simulink model "Final_EWASP_VC"  (R2022a)
settings: Solver=ode1  StartTime=0.0  StopTime=24*3600  FixedStep=10  RelTol=1e-3
values from neighbouring files (symbols this model uses):
  Aux_Threshold = 52    [Setup_Code_EWASP_VC.m]
  buildingAge = 2005    [Setup_Code_EWASP_VC.m]
  ceilingHeight = 2.4    [Setup_Code_EWASP_VC.m]
  conductiveHconnectMatrix = [ ... (first row only)    [Setup_Code_EWASP_VC.m]
  cRoofGreen = 100000    [Setup_Code_EWASP_VC.m]
  Defrost_After_Time = 30    [Setup_Code_EWASP_VC.m]
  DHWDemandProfile = occFreegainHotwaterElecTestPassiveOcc3(:,3)    [Setup_Code_EWASP_VC.m]
  Elec_Max = Elec_Max*(30/24.2)    [Setup_Code_EWASP_VC.m]
  Elec_Mid = Elec_Mid*(30/24.2)    [Setup_Code_EWASP_VC.m]
  Elec_Min = Elec_Min*(30/24.2)    [Setup_Code_EWASP_VC.m]
  ElecDemandProfile = occFreegainHotwaterElecTestPassiveOcc3(:,4)    [Setup_Code_EWASP_VC.m]
  ElecFixed = [Elec_Max(6,2) Elec_Max(6,4) Elec_Max(6,6) Elec_Max(6,7) ... (first row only)    [Setup_Code_EWASP_VC.m]
  floorOrCeilingArea = floorOrCeilingArea*1.15    [Setup_Code_EWASP_VC.m]
  forceCold = 0    [Setup_Code_EWASP_VC.m]
  freegain = occFreegainHotwaterElecTestPassiveOcc3(:,2)-max(occupancy)*25    [Setup_Code_EWASP_VC.m]
  furnitureModelOn = 1    [Setup_Code_EWASP_VC.m]
  Heat_Max = Heat_Max*(30/24.2)    [Setup_Code_EWASP_VC.m]
  Heat_Mid = Heat_Mid*(30/24.2)    [Setup_Code_EWASP_VC.m]
  Heat_Min = Heat_Min*(30/24.2)    [Setup_Code_EWASP_VC.m]
  HeatFixed = [Heat_Max(6,2) Heat_Max(6,4) Heat_Max(6,6) Heat_Max(6,7) ... (first row only)    [Setup_Code_EWASP_VC.m]
  HeatingOnProfile = repmat(HeatingOnProfile,365,1)    [Setup_Code_EWASP_VC.m]
  HEX_ReturnLowerLimit = 52.5    [Setup_Code_EWASP_VC.m]
  HEX_ReturnUpperLimit = 55    [Setup_Code_EWASP_VC.m]
  LeakMultiplier = 1+(2*(rand()-0.5)/10)    [Setup_Code_EWASP_VC.m]
  loopCap = 15    [Setup_Code_EWASP_VC.m]
  maxOcc = max(occupancyProfile)    [Setup_Code_EWASP_VC.m]
  NESW_wallArea = max(NESW_Lengths*ceilingHeight-NESW_Windows,0)    [Setup_Code_EWASP_VC.m]
  NESW_Windows = [ ... (first row only)    [Setup_Code_EWASP_VC.m]
  numRooms = roomCount    [Setup_Code_EWASP_VC.m]
  offsetDays = 0    [Setup_Code_EWASP_VC.m]
  pumpChoice = pumpChoices(MinIndex,1)    [Setup_Code_EWASP_VC.m]
  pumpRamp = 180    [Setup_Code_EWASP_VC.m]
  ReturnLowerLimit = 37.5    [Setup_Code_EWASP_VC.m]
  ReturnUpperLimit = 40    [Setup_Code_EWASP_VC.m]
  RoofIrradiance = Flat_NS_EW_RoofIrradiance(:,1)    [Setup_Code_EWASP_VC.m]
  roofStartTemp = ones(11,1)*20    [Setup_Code_EWASP_VC.m]
  rooftype = 0    [Setup_Code_EWASP_VC.m]
  RoomDataMatrix = [zeros(1,12);ones(1,12)*wallDensity;zeros(1,12);ones(1,12)*wallU;ones(1,12)*windowU;ones(1,12)*floorU;ones(1,12)*ceilingU;zeros(1,12);windowArea, 0;floorOrCeilingArea;zeros(1,12);floorOrCeilingArea*ceilingHeight]    [Setup_Code_EWASP_VC.m]
  roomVol = roomVol*1.15    [Setup_Code_EWASP_VC.m]
  slabStartTemp = (GroundTempTimeSeries(offsetDays*1440+1,1)+thermostatSetting)/2    [Setup_Code_EWASP_VC.m]
  SlackRequest = zeros(1440,1)    [Setup_Code_EWASP_VC.m]
  SolarThermalExists = 0    [Setup_Code_EWASP_VC.m]
  SourceFixed = HeatFixed-ElecFixed    [Setup_Code_EWASP_VC.m]
  StateSeries = StateSeriesGenerator(22,7,1)    [Setup_Code_EWASP_VC.m]
  Tank_Lower_Temp = 49.5    [Setup_Code_EWASP_VC.m]
  Tank_Upper_Temp = 52    [Setup_Code_EWASP_VC.m]
  Tank_Volume_m3 = 0.15    [Setup_Code_EWASP_VC.m]
  TankHeatHour = randi([1 5])-1    [Setup_Code_EWASP_VC.m]
  thermostatSetting = 20.0    (= 20)    [Setup_Code_EWASP_VC.m]
  upDown = [0;0;0;0;1;1;1;1;1;1;1]    [Setup_Code_EWASP_VC.m]
  variableASHP = 1    [Setup_Code_EWASP_VC.m]
  wallStartTempExt = thermostatSetting*(0.266+0.00215*outdoorStartTemp+0.018*wallU+0.00113*outdoorStartTemp*wallU+0.0068*wallU^2)    [Setup_Code_EWASP_VC.m]
undefined symbols (not defined in the file or in its folder): a, ceilingU, condUDMatrix, convUDMatrix, deltaPEXPANDED_E, deltaPEXPANDED_E2, deltaPEXPANDED_N, deltaPEXPANDED_N2, deltaPEXPANDED_S, deltaPEXPANDED_S2, deltaPEXPANDED_W, deltaPEXPANDED_W2, DesiredDHWTemp, DesiredFlowTempVsInOutDeltaTemp, DiffuseHorizontal, DiscIntNeverNeededParam, DNI, dwnAndConcrete, DWORK_A_HX, DWORK_CHK_FLU, DWORK_CP_NODE, DWORK_DH, DWORK_FLUID, DWORK_HCON, DWORK_LOSS, DWORK_MDOTDOWN, DWORK_MDOTIN, DWORK_MDOTUP, DWORK_MIX, DWORK_PRESS, DWORK_QDOTIN, DWORK_RHO_NODE, DWORK_TIN, DWORK_TS_OLD, DWORK_V_NODE, GroundTempTimeSeries, HCM, HCM2, HCM_closed, HCM_closed2, intermediateU, IsTop, massFlowMatrix, neighbourMatrix, numericalRoomUse, RadiatorMatrix, room2roomflowmatrix_E, room2roomflowmatrix_E2, room2roomflowmatrix_N, room2roomflowmatrix_N2, room2roomflowmatrix_S, room2roomflowmatrix_S2, room2roomflowmatrix_W, room2roomflowmatrix_W2, StateAirInEXPANDED_E, StateAirInEXPANDED_E2, StateAirInEXPANDED_N, StateAirInEXPANDED_N2, StateAirInEXPANDED_S, StateAirInEXPANDED_S2 ... (+23)
libraries: simulink x6, dspsigops x4, dspmtrx3 x4, carnot x3, spsEdgeDetectorLib x2, dspstat3 x2, powerlib_meascontrol x1, simulink_extras x1
(part 2 of 27)

== system Final_EWASP_VC/GSHP_Subsystem ==
  note: Monitors for debugging
  Constant3 : Constant  Value=3600
  DHW for GSHP case : Subsystem
  Delay6 : Delay  DelayLength=5  InitialCondition=0
  Discrete-Time Integrator1 : DiscreteIntegrator  ExternalReset=falling  SampleTime=-1  LimitOutput=on  UpperSaturationLimit=1  LowerSaturationLimit=0  ICPrevOutput=DiscIntNeverNeededParam  ICPrevScaledInput=DiscIntNeverNeededParam
  Divide1 : Product  Inputs=*/
  Divide2 : Product  Inputs=*/
  Integrator14 : Integrator
  IsInf : RelationalOperator  Operator=isNaN  OutDataTypeStr=boolean  RndMeth=Simplest  InputSameDT=off
  Massflow when system is on12 : Constant  Value=3400/3600
  Plus : Sum
  Product : Product
  Product1 : Product
  Product3 : Product  Inputs=*/
  Scope21 : Scope
  Subsystem3 : Subsystem
      mask Display:
      | port_label('input', 1, 'T_Out')
      | port_label('input', 2, 'MixedTemp')
      | port_label('input', 3, 'MassFlowTotal')
      | port_label('input', 4, 'GCS')
      | port_label('input', 5, 'PowerFraction')
      | port_label('input', 6, 'DHW_on')
      | port_label('input', 7, 'ToGroundTot')
      | 
      | port_label('output', 1, 'Hysteresis')
      | port_label('output', 2, 'd_signal')
      | port_label('output', 3, 'THB_to_Pre')
      | 
      | port_label('output', 4, 'HeatToSpace')
      | port_label('output', 5, 'ElectrifiedHeatToSpace')
      | port_label('output', 6, 'ToGround')
      | port_label('output', 7, 'TotMdot')
      | 
      | disp('SH_GSHP')
  Sum : Sum  Inputs=|++
  Sum7 : Sum  Inputs=|++
  Switch2 : Switch  Criteria=u2 > Threshold  Threshold=0.5  SaturateOnIntegerOverflow=off  InputSameDT=off
  T_mains : Constant  Value=12
  Time in seconds for Heat pump to reach full stady state output1 : Constant  Value=180
  Water Demand Time Series (Minute)1 : Constant  Value=DHWDemandProfile
  tank_sensor_temp : Scope
  tag scope: AuxHeatToWater=global, DHW_on=global, ElectrifiedHeatToSpaceG=global, ElectrifiedHeatToWater=global, HeatToSpace=global, HeatToWater=global, THB_In_Pre=global, ToGround2=global, ToGround=global, ToGroundTot=global, TotMdot2=global, TotMdot=global, d_signal=global, d_signal_DHW=global, hysteresis=global, pump_power_Fraction=global
  wires:
  Product3/1 -> Switch2/3, IsInf/1
  Water Demand Time Series (Minute)1/1 -> DHW for GSHP case/5(In5)
  Subsystem3/4(Out4) -> [HeatToSpace]
  Integrator14/1 -> Scope21/1
  Divide2/1 -> Discrete-Time Integrator1/1
  DHW for GSHP case/1(Out1) -> tank_sensor_temp/1
  [d_signal] -> Plus/1
  DHW for GSHP case/2(Out2) -> [DHW_on]
  [MassFlowTotal] -> Subsystem3/3(In3)
  [DHW_on] -> Subsystem3/6(In6)
  [T_Out] -> Subsystem3/1(In1)
  DHW for GSHP case/7(Out7) -> [AuxHeatToWater]
  Discrete-Time Integrator1/1 -> Delay6/1
  [ToGround] -> Switch2/1, Product/1
  DHW for GSHP case/6(Out6) -> [HeatToWater]
  Subsystem3/3(Out3) -> [THB_In_Pre]
  [MixedTemp] -> Subsystem3/2(In2)
  Subsystem3/1(Out1) -> [hysteresis]
  [FromGround] -> DHW for GSHP case/1(In1)
  Plus/1 -> Divide2/1, Discrete-Time Integrator1/2
  Time in seconds for Heat pump to reach full stady state output1/1 -> Divide2/2
  [ToGround2] -> Product1/1
  [HeatToSpace] -> Divide1/1
  DHW for GSHP case/3(Out3) -> [ToGround2]
  [d_signal_DHW] -> Plus/2
  DHW for GSHP case/5(Out5) -> [ElectrifiedHeatToWater]
  Delay6/1 -> [pump_power_Fraction]
  Divide1/1 -> Integrator14/1
  [TotMdot] -> Product/2, Sum/1
  Product/1 -> Sum7/1
  DHW for GSHP case/4(Out4) -> [TotMdot2]
  Constant3/1 -> Divide1/2
  Subsystem3/7(Out7) -> [TotMdot]
  Massflow when system is on12/1 -> DHW for GSHP case/6(In6)
  DHW for GSHP case/8(Out8) -> [d_signal_DHW]
  [pump_power_Fraction] -> Subsystem3/5(In5)
  Subsystem3/6(Out6) -> [ToGround]
  Subsystem3/5(Out5) -> [ElectrifiedHeatToSpaceG]
  [ToGroundTot] -> Subsystem3/7(In7)
  Subsystem3/2(Out2) -> [d_signal]
  [Global_Control_Signal] -> Subsystem3/4(In4)
  [TotMdot2] -> Product1/2, Sum/2
  Sum/1 -> Product3/2
  [T_Out] -> DHW for GSHP case/3(In3)
  Product1/1 -> Sum7/2
  Sum7/1 -> Product3/1
  T_mains/1 -> DHW for GSHP case/4(In4)
  IsInf/1 -> Switch2/2
  Switch2/1 -> [ToGroundTot]
  [T_1] -> DHW for GSHP case/2(In2)
  Subsystem3/8(Out8) -> [FromGround]

== system Final_EWASP_VC/Offset Independent time series element selector ==
  In1 : Inport
  Clock1 : Clock
  Direct Lookup Table (n-D)1 : LookupNDDirect  NumberOfTableDimensions=1  TableIsInput=on
  Divide1 : Product  Inputs=*/
  Floor : Rounding
  Saturation2 : Saturate  UpperLimit=inf  LowerLimit=0
  Scope23 : Scope
  Sum : Sum  Inputs=|++
  on? (I/O)1 : Constant  Value=0  OutDataTypeStr=double
  on? (I/O)3 : Constant  Value=60  OutDataTypeStr=double
  Out1 : Outport  VectorParamsAs1DForOutWhenUnconnected=off
  wires:
  Saturation2/1 -> Scope23/1, Direct Lookup Table (n-D)1/1
  on? (I/O)3/1 -> Divide1/2
  Divide1/1 -> Floor/1
  Floor/1 -> Saturation2/1
  Clock1/1 -> Sum/1
  Direct Lookup Table (n-D)1/1 -> Out1/1
  In1/1 -> Direct Lookup Table (n-D)1/2
  on? (I/O)1/1 -> Sum/2
  Sum/1 -> Divide1/1

== system Final_EWASP_VC/Offset Independent time series element selector1 ==
  In1 : Inport
  Clock1 : Clock
  Direct Lookup Table (n-D)1 : LookupNDDirect  NumberOfTableDimensions=1  TableIsInput=on
  Divide1 : Product  Inputs=*/
  Floor : Rounding
  Saturation2 : Saturate  UpperLimit=inf  LowerLimit=0
  Scope23 : Scope
  Sum : Sum  Inputs=|++
  on? (I/O)2 : Constant  Value=offsetDays*3600*24  OutDataTypeStr=double
  on? (I/O)3 : Constant  Value=60  OutDataTypeStr=double
  Out1 : Outport  VectorParamsAs1DForOutWhenUnconnected=off
  wires:
  Saturation2/1 -> Scope23/1, Direct Lookup Table (n-D)1/1
  on? (I/O)3/1 -> Divide1/2
  Divide1/1 -> Floor/1
  Floor/1 -> Saturation2/1
  Clock1/1 -> Sum/1
  Direct Lookup Table (n-D)1/1 -> Out1/1
  In1/1 -> Direct Lookup Table (n-D)1/2
  Sum/1 -> Divide1/1
  on? (I/O)2/1 -> Sum/2

== system Final_EWASP_VC/Offset Independent time series element selector2 ==
  In1 : Inport
  Clock1 : Clock
  Direct Lookup Table (n-D)1 : LookupNDDirect  NumberOfTableDimensions=1  TableIsInput=on
  Divide1 : Product  Inputs=*/
  Floor : Rounding
  Saturation2 : Saturate  UpperLimit=inf  LowerLimit=0
  Scope23 : Scope
  Sum : Sum  Inputs=|++
  on? (I/O)1 : Constant  Value=0  OutDataTypeStr=double
  on? (I/O)3 : Constant  Value=60  OutDataTypeStr=double
  Out1 : Outport  VectorParamsAs1DForOutWhenUnconnected=off
  wires:
  Saturation2/1 -> Scope23/1, Direct Lookup Table (n-D)1/1
  on? (I/O)3/1 -> Divide1/2
  Divide1/1 -> Floor/1
  Floor/1 -> Saturation2/1
  Clock1/1 -> Sum/1
  Direct Lookup Table (n-D)1/1 -> Out1/1
  In1/1 -> Direct Lookup Table (n-D)1/2
  on? (I/O)1/1 -> Sum/2
  Sum/1 -> Divide1/1

== system Final_EWASP_VC/Radiator w//Thermostatic Control ==
  In1 : Inport
  In2 : Inport  Port=2
  In3 : Inport  Port=3
  1/(m*cp) : Gain  Gain=1/(Water_Volume*4180)  SaturateOnIntegerOverflow=on  OutDataTypeStr=Inherit: Same as input  ParamDataTypeStr=Inherit: Same as input
  Abs : Abs
  Add : Sum  Inputs=+-
  Constant : Constant  Value=4181
  Constant1 : Constant  Value=TRV_Therm_Setpoint
  Constant2 : Constant  Value=0.5
  Discrete-Time Integrator : DiscreteIntegrator  SampleTime=-1  ICPrevOutput=DiscIntNeverNeededParam  ICPrevScaledInput=DiscIntNeverNeededParam
  Divide : Product  Inputs=*/
  Divide1 : Product  Inputs=**
  Math Function : Math  Operator=pow  SignedPower=on
  Product : Product  Inputs=3  InputSameDT=on  SaturateOnIntegerOverflow=on  OutDataTypeStr=Inherit: Same as first input
  Product1 : Product  InputSameDT=on  SaturateOnIntegerOverflow=on  OutDataTypeStr=Inherit: Same as first input
  Product2 : Product
  Qdot2room1 : Scope
  Saturation : Saturate  UpperLimit=1  LowerLimit=0
  Scope : Scope
  Sign : Signum
  Sum : Sum  Inputs=-+  InputSameDT=on  SaturateOnIntegerOverflow=on  OutDataTypeStr=Inherit: Same as first input
  Sum1 : Sum  Inputs=-+  InputSameDT=on  SaturateOnIntegerOverflow=on  OutDataTypeStr=Inherit: Same as first input
  Sum2 : Sum
  Sum3 : Sum  Inputs=-+  InputSameDT=on  SaturateOnIntegerOverflow=on  OutDataTypeStr=Inherit: Same as first input
  Transfer Fcn (with initial states) : simulink_extras/Additional Linear/Transfer Fcn (with initial states)  Commented=on  N=[1]  D="[1  0]"  X0=20
  const : Constant  Value=1.3
  const1 : Constant  Value=Power_Nominal
  dTnom : Constant  Value=DeltaT_Nominal
  Out1 : Outport  VectorParamsAs1DForOutWhenUnconnected=off
  Out2 : Outport  Port=2  VectorParamsAs1DForOutWhenUnconnected=off
  Out3 : Outport  Port=3  VectorParamsAs1DForOutWhenUnconnected=off
  wires:
  Sum/1 -> Product/1
  Sum1/1 -> 1/(m*cp)/1
  Constant/1 -> Product/3
  Sum3/1 -> Sign/1, Divide/1
  const/1 -> Math Function/2
  Sign/1 -> Product1/2
  Product1/1 -> Out1/1, Sum1/1
  dTnom/1 -> Divide/2
  Abs/1 -> Math Function/1
  Product/1 -> Sum1/2
  In2/1 -> Sum/2
  const1/1 -> Divide1/2
  Divide1/1 -> Product1/1
  1/(m*cp)/1 -> Discrete-Time Integrator/1
  Math Function/1 -> Divide1/1
  Discrete-Time Integrator/1 -> Sum3/2, Sum/1, Scope/1, Out2/1
  Divide/1 -> Abs/1
  In1/1 -> Add/2, Sum3/1
  Product2/1 -> Product/2, Out3/1
  In3/1 -> Product2/1
  Constant1/1 -> Add/1
  Add/1 -> Sum2/1
  Constant2/1 -> Sum2/2
  Sum2/1 -> Saturation/1
  Saturation/1 -> Qdot2room1/1, Product2/2

== system Final_EWASP_VC/Select Correct Element from Array1 ==
  In1 : Inport
  Constant : Constant  Value=60
  Digital Clock : DigitalClock  SampleTime=10
  Direct Lookup Table (n-D) : LookupNDDirect  NumberOfTableDimensions=1  TableIsInput=on
  Divide : Product  Inputs=*/
  Floor : Rounding
  Saturation : Saturate  UpperLimit=inf  LowerLimit=0
  Out1 : Outport  VectorParamsAs1DForOutWhenUnconnected=off
  wires:
  Divide/1 -> Floor/1
  Saturation/1 -> Direct Lookup Table (n-D)/1
  Constant/1 -> Divide/2
  Floor/1 -> Saturation/1
  In1/1 -> Direct Lookup Table (n-D)/2
  Digital Clock/1 -> Divide/1
  Direct Lookup Table (n-D)/1 -> Out1/1

== system Final_EWASP_VC/Select Correct Element from Array2 ==
  In1 : Inport
  Constant : Constant  Value=60
  Digital Clock : DigitalClock  SampleTime=10
  Direct Lookup Table (n-D) : LookupNDDirect  NumberOfTableDimensions=1  TableIsInput=on
  Divide : Product  Inputs=*/
  Floor : Rounding
  Saturation : Saturate  UpperLimit=1439  LowerLimit=0
  Out1 : Outport  VectorParamsAs1DForOutWhenUnconnected=off
  wires:
  Divide/1 -> Floor/1
  Saturation/1 -> Direct Lookup Table (n-D)/1
  Constant/1 -> Divide/2
  Floor/1 -> Saturation/1
  In1/1 -> Direct Lookup Table (n-D)/2
  Digital Clock/1 -> Divide/1
  Direct Lookup Table (n-D)/1 -> Out1/1

== system Final_EWASP_VC/Select correct element from array, considering offset ==
  In1 : Inport
  Clock1 : Clock
  Direct Lookup Table (n-D)1 : LookupNDDirect  NumberOfTableDimensions=1  TableIsInput=on
  Divide1 : Product  Inputs=*/
  Floor : Rounding
  Saturation2 : Saturate  UpperLimit=inf  LowerLimit=0
  Scope23 : Scope
  Sum : Sum  Inputs=|++
  on? (I/O)1 : Constant  Value=offsetDays*3600*24  OutDataTypeStr=double
  on? (I/O)3 : Constant  Value=60  OutDataTypeStr=double
  Out1 : Outport  VectorParamsAs1DForOutWhenUnconnected=off
  wires:
  Saturation2/1 -> Scope23/1, Direct Lookup Table (n-D)1/1
  on? (I/O)3/1 -> Divide1/2
  Divide1/1 -> Floor/1
  Floor/1 -> Saturation2/1
  Clock1/1 -> Sum/1
  Direct Lookup Table (n-D)1/1 -> Out1/1
  In1/1 -> Direct Lookup Table (n-D)1/2
  on? (I/O)1/1 -> Sum/2
  Sum/1 -> Divide1/1

== system Final_EWASP_VC/Select correct element from array, considering offset1 ==
  In1 : Inport
  Clock1 : Clock
  Direct Lookup Table (n-D)1 : LookupNDDirect  NumberOfTableDimensions=1  TableIsInput=on
  Divide1 : Product  Inputs=*/
  Floor : Rounding
  Saturation2 : Saturate  UpperLimit=inf  LowerLimit=0
  Scope23 : Scope
  Sum : Sum  Inputs=|++
  on? (I/O)1 : Constant  Value=offsetDays*3600*24  OutDataTypeStr=double
  on? (I/O)3 : Constant  Value=60  OutDataTypeStr=double
  Out1 : Outport  VectorParamsAs1DForOutWhenUnconnected=off
  wires:
  Saturation2/1 -> Scope23/1, Direct Lookup Table (n-D)1/1
  on? (I/O)3/1 -> Divide1/2
  Divide1/1 -> Floor/1
  Floor/1 -> Saturation2/1
  Clock1/1 -> Sum/1
  Direct Lookup Table (n-D)1/1 -> Out1/1
  In1/1 -> Direct Lookup Table (n-D)1/2
  on? (I/O)1/1 -> Sum/2
  Sum/1 -> Divide1/1

== system Final_EWASP_VC/Select correct element from array, considering offset2 ==
  In1 : Inport
  Clock1 : Clock
  Direct Lookup Table (n-D)1 : LookupNDDirect  NumberOfTableDimensions=1  TableIsInput=on
  Divide1 : Product  Inputs=*/
  Floor : Rounding
  Saturation2 : Saturate  UpperLimit=inf  LowerLimit=0
  Scope23 : Scope
  Sum : Sum  Inputs=|++
  on? (I/O)1 : Constant  Value=offsetDays*3600*24  OutDataTypeStr=double
  on? (I/O)3 : Constant  Value=60  OutDataTypeStr=double
  Out1 : Outport  VectorParamsAs1DForOutWhenUnconnected=off
  wires:
  Saturation2/1 -> Scope23/1, Direct Lookup Table (n-D)1/1
  on? (I/O)3/1 -> Divide1/2
  Divide1/1 -> Floor/1
  Floor/1 -> Saturation2/1
  Clock1/1 -> Sum/1
  Direct Lookup Table (n-D)1/1 -> Out1/1
  In1/1 -> Direct Lookup Table (n-D)1/2
  on? (I/O)1/1 -> Sum/2
  Sum/1 -> Divide1/1

== system Final_EWASP_VC/Select correct element from array, considering offset3 ==
  In1 : Inport
  Clock1 : Clock
  Direct Lookup Table (n-D)1 : LookupNDDirect  NumberOfTableDimensions=1  TableIsInput=on
  Divide1 : Product  Inputs=*/
  Floor : Rounding
  Saturation2 : Saturate  UpperLimit=inf  LowerLimit=0
  Scope23 : Scope
  Sum : Sum  Inputs=|++
  on? (I/O)1 : Constant  Value=offsetDays*3600*24  OutDataTypeStr=double
  on? (I/O)3 : Constant  Value=60  OutDataTypeStr=double
  Out1 : Outport  VectorParamsAs1DForOutWhenUnconnected=off
  wires:
  Saturation2/1 -> Scope23/1, Direct Lookup Table (n-D)1/1
  on? (I/O)3/1 -> Divide1/2
  Divide1/1 -> Floor/1
  Floor/1 -> Saturation2/1
  Clock1/1 -> Sum/1
  Direct Lookup Table (n-D)1/1 -> Out1/1
  In1/1 -> Direct Lookup Table (n-D)1/2
  on? (I/O)1/1 -> Sum/2
  Sum/1 -> Divide1/1

== system Final_EWASP_VC/Select correct element from array, considering offset4 ==
  In1 : Inport
  Clock1 : Clock
  Direct Lookup Table (n-D)1 : LookupNDDirect  NumberOfTableDimensions=1  TableIsInput=on
  Divide1 : Product  Inputs=*/
  Floor : Rounding
  Saturation2 : Saturate  UpperLimit=inf  LowerLimit=0
  Scope23 : Scope
  Sum : Sum  Inputs=|++
  on? (I/O)1 : Constant  Value=offsetDays*3600*24  OutDataTypeStr=double
  on? (I/O)3 : Constant  Value=60  OutDataTypeStr=double
  Out1 : Outport  VectorParamsAs1DForOutWhenUnconnected=off
  wires:
  Saturation2/1 -> Scope23/1, Direct Lookup Table (n-D)1/1
  on? (I/O)3/1 -> Divide1/2
  Divide1/1 -> Floor/1
  Floor/1 -> Saturation2/1
  Clock1/1 -> Sum/1
  Direct Lookup Table (n-D)1/1 -> Out1/1
  In1/1 -> Direct Lookup Table (n-D)1/2
  on? (I/O)1/1 -> Sum/2
  Sum/1 -> Divide1/1

== system Final_EWASP_VC/Subsystem ==
  note: Bodged here - need to get a code that finds last non nan value
  In1 : Inport
  In2 : Inport  Port=2
  In3 : Inport  Port=3
  In4 : Inport  Port=4
  In5 : Inport  Port=5
  In6 : Inport  Port=6
  In7 : Inport  Port=7
  In8 : Inport  Port=8
  In9 : Inport  Port=9
  In10 : Inport  Port=10
  In11 : Inport  Port=11
  In12 : Inport  Port=12
  In13 : Inport  Port=13
  In14 : Inport  Port=14
  In15 : Inport  Port=15
  In16 : Inport  Port=16
  In17 : Inport  Port=17
  In18 : Inport  Port=18
  In19 : Inport  Port=19
  In20 : Inport  Port=20
  In21 : Inport  Port=21
  In22 : Inport  Port=22
  In23 : Inport  Port=23
  In24 : Inport  Port=24
  Add{1..4} (4 alike) : Sum  Inputs=12
  Ceil{,1..11} (12 alike) : Rounding  Operator=ceil
  Connect Count1 : Display
  Constant : Constant  Value=11
  Divide : Product  Inputs=*/
  IsNaN : RelationalOperator  Operator=isNaN  OutDataTypeStr=boolean  RndMeth=Simplest  InputSameDT=off
  "MassFlow. " : Display
  Product{,1..11} (12 alike) : Product
  Scope : Scope
  Scope1 : Scope
  Switch5 : Switch  Criteria=u2 > Threshold  Threshold=0.5  SaturateOnIntegerOverflow=off  InputSameDT=off
  positive delta T2 : Product  Inputs=*/
  Out1 : Outport  VectorParamsAs1DForOutWhenUnconnected=off
  Out2 : Outport  Port=2  VectorParamsAs1DForOutWhenUnconnected=off
  wires:
  Product5/1 -> Add2/6
  Product/1 -> Add2/1
  [SumUp12] -> Product11/1
  [SumUp9] -> Product8/1
  [SumUp9] -> Add1/9
  [SumUp7] -> Product6/1
  Product9/1 -> Add2/10
  [SumUp5] -> Product4/1
  [SumUp3] -> Add1/3
  In14/1 -> Add3/2, Product1/2
  In20/1 -> Add3/8, Product7/2
  Product8/1 -> Add2/9
  positive delta T2/1 -> Scope1/1, Switch5/3, Connect Count1/1, IsNaN/1
  [SumUp5] -> Add1/5
  Product1/1 -> Add2/2
  Product10/1 -> Add2/11
  [SumUp3] -> Product2/1
  Product6/1 -> Add2/7
  In15/1 -> Product2/2, Add3/3
  [SumUp4] -> Add1/4
  In17/1 -> Product4/2, Add3/5
  [SumUp2] -> Product1/1
  Add1/1 -> positive delta T2/2, Out1/1, "MassFlow. "/1
  In10/1 -> [SumUp10]
  [SumUp] -> Product/1
  [SumUp6] -> Product5/1
  In2/1 -> [SumUp2]
  Product4/1 -> Add2/5
  [SumUp6] -> Add1/6
  In24/1 -> Product11/2, Add3/12
  [SumUp11] -> Product10/1
  Product7/1 -> Add2/8
  Product3/1 -> Add2/4
  In18/1 -> Product5/2, Add3/6
  [SumUp7] -> Add1/7
  Product11/1 -> Add2/12
  [SumUp4] -> Product3/1
  In7/1 -> [SumUp7]
  Product2/1 -> Add2/3
  In23/1 -> Add3/11, Product10/2
  [SumUp11] -> Add1/11
  In16/1 -> Add3/4, Product3/2
  [SumUp10] -> Product9/1
  [SumUp12] -> Add1/12
  [SumUp10] -> Add1/10
  [SumUp2] -> Add1/2
  [SumUp] -> Add1/1
  In9/1 -> [SumUp9]
  [SumUp8] -> Product7/1
  In22/1 -> Product9/2, Add3/10
  Add2/1 -> positive delta T2/1
  [SumUp8] -> Add1/8
  In12/1 -> [SumUp12]
  In11/1 -> [SumUp11]
  In6/1 -> [SumUp6]
  In8/1 -> [SumUp8]
  In21/1 -> Add3/9, Product8/2
  In13/1 -> Add3/1, Product/2
  In19/1 -> Product6/2, Add3/7
  In5/1 -> [SumUp5]
  In3/1 -> [SumUp3]
  In4/1 -> [SumUp4]
  In1/1 -> [SumUp]
  Divide/1 -> Switch5/1
  IsNaN/1 -> Switch5/2
  Switch5/1 -> Out2/1
  Add3/1 -> Divide/1
  Constant/1 -> Divide/2
  [SumUp] -> Ceil/1
  [SumUp2] -> Ceil1/1
  [SumUp3] -> Ceil2/1
  [SumUp4] -> Ceil3/1
  [SumUp5] -> Ceil4/1
  [SumUp6] -> Ceil5/1
  [SumUp7] -> Ceil6/1
  [SumUp8] -> Ceil7/1
  [SumUp9] -> Ceil8/1
  [SumUp10] -> Ceil9/1
  [SumUp11] -> Ceil10/1
  [SumUp12] -> Ceil11/1
  Ceil/1 -> Add4/1
  Ceil1/1 -> Add4/2
  Ceil2/1 -> Add4/3
  Ceil3/1 -> Add4/4
  Ceil4/1 -> Add4/5
  Ceil5/1 -> Add4/6
  Ceil6/1 -> Add4/7
  Ceil7/1 -> Add4/8
  Ceil8/1 -> Add4/9
  Ceil9/1 -> Add4/10
  Ceil10/1 -> Add4/11
  Ceil11/1 -> Add4/12
  Add4/1 -> Scope/1

== system Final_EWASP_VC/Subsystem1 ==
  In1 : Inport
  In2 : Inport  Port=2
  In3 : Inport  Port=3
  In4 : Inport  Port=4
  In5 : Inport  Port=5
  In6 : Inport  Port=6
  In7 : Inport  Port=7
  In8 : Inport  Port=8
  In9 : Inport  Port=9
  In10 : Inport  Port=10
  In11 : Inport  Port=11
  In12 : Inport  Port=12
  In13 : Inport  Port=13
  Massflow when system is off{3..14} (12 alike) : Constant  Value=0
  Switch{7..18} (12 alike) : Switch  Criteria=u2 > Threshold  Threshold=0.5  SaturateOnIntegerOverflow=off  InputSameDT=off
  Out1 : Outport  VectorParamsAs1DForOutWhenUnconnected=off
  Out2 : Outport  Port=2  VectorParamsAs1DForOutWhenUnconnected=off
  Out3 : Outport  Port=3  VectorParamsAs1DForOutWhenUnconnected=off
  Out4 : Outport  Port=4  VectorParamsAs1DForOutWhenUnconnected=off
  Out5 : Outport  Port=5  VectorParamsAs1DForOutWhenUnconnected=off
  Out6 : Outport  Port=6  VectorParamsAs1DForOutWhenUnconnected=off
  Out7 : Outport  Port=7  VectorParamsAs1DForOutWhenUnconnected=off
  Out8 : Outport  Port=8  VectorParamsAs1DForOutWhenUnconnected=off
  Out9 : Outport  Port=9  VectorParamsAs1DForOutWhenUnconnected=off
  Out10 : Outport  Port=10  VectorParamsAs1DForOutWhenUnconnected=off
  Out11 : Outport  Port=11  VectorParamsAs1DForOutWhenUnconnected=off
  Out12 : Outport  Port=12  VectorParamsAs1DForOutWhenUnconnected=off
  wires:
  Massflow when system is off10/1 -> Switch11/3
  Switch9/1 -> Out3/1
  Switch7/1 -> Out1/1
  In1/1 -> Switch7/2, Switch9/2, Switch10/2, Switch17/2, Switch15/2, Switch18/2, Switch16/2, Switch11/2, Switch14/2, Switch13/2, Switch12/2, Switch8/2
  Massflow when system is off5/1 -> Switch9/3
  In4/1 -> Switch9/1
  Massflow when system is off6/1 -> Switch10/3
  Switch11/1 -> Out8/1
  Switch14/1 -> Out7/1
  Massflow when system is off11/1 -> Switch16/3
  Massflow when system is off9/1 -> Switch14/3
  Massflow when system is off13/1 -> Switch18/3
  Switch15/1 -> Out12/1
  Switch10/1 -> Out4/1
  Switch17/1 -> Out10/1
  Massflow when system is off3/1 -> Switch7/3
  Massflow when system is off4/1 -> Switch8/3
  Massflow when system is off14/1 -> Switch15/3
  In12/1 -> Switch18/1
  Massflow when system is off12/1 -> Switch17/3
  In7/1 -> Switch13/1
  Switch12/1 -> Out5/1
  In5/1 -> Switch10/1
  Massflow when system is off8/1 -> Switch13/3
  Massflow when system is off7/1 -> Switch12/3
  In11/1 -> Switch17/1
  Switch18/1 -> Out11/1
  In9/1 -> Switch11/1
  Switch13/1 -> Out6/1
  In3/1 -> Switch8/1
  In2/1 -> Switch7/1
  Switch16/1 -> Out9/1
  In13/1 -> Switch15/1
  In10/1 -> Switch16/1
  In6/1 -> Switch12/1
  In8/1 -> Switch14/1
  Switch8/1 -> Out2/1

== system Final_EWASP_VC/Subsystem2 ==
  note: last off
  In1 : Inport
  Clock : Clock
  Clock1 : Clock
  Clock3 : Clock
  Delay1 : Delay  DelayLength=1  InitialCondition=0
  Delay2 : Delay  DelayLength=1  InitialCondition=0
  Ground : Ground
  Logical Operator1 : Logic  AllPortsSameDT=off  OutDataTypeStr=boolean
  Logical Operator2 : Logic  Operator=NOT  AllPortsSameDT=off  OutDataTypeStr=boolean
  Logical Operator3 : Logic  AllPortsSameDT=off  OutDataTypeStr=boolean
  Logical Operator4 : Logic  Operator=NOT  AllPortsSameDT=off  OutDataTypeStr=boolean
  Memory : Memory
  Sample and Hold : dspsigops/Sample and Hold  trig=Rising edge  initCond=0  latchinput=off
  Sample and Hold1 : dspsigops/Sample and Hold  trig=Rising edge  initCond=0  latchinput=off
  Scope20 : Scope  NumInputPorts=2
  Scope21 : Scope
  Subtract : Sum  Inputs=-+
  Subtract1 : Sum  Inputs=+-
  Switch2 : Switch  Criteria=u2 > Threshold  SaturateOnIntegerOverflow=off  InputSameDT=off
  Switch3 : Switch  Threshold=1  SaturateOnIntegerOverflow=off  InputSameDT=off
  Switch4 : Switch  Criteria=u2 > Threshold  Threshold=600  SaturateOnIntegerOverflow=off  InputSameDT=off
  on? (I/O)3 : Constant  OutDataTypeStr=double
  on? (I/O)4 : Constant  Value=0  OutDataTypeStr=double
  on? (I/O)5 : Constant  OutDataTypeStr=double
  on? (I/O)6 : Constant  OutDataTypeStr=double
  on? (I/O)7 : Constant  Value=0  OutDataTypeStr=double
  Out1 : Outport  VectorParamsAs1DForOutWhenUnconnected=off
  wires:
  Clock3/1 -> Sample and Hold/1
  Sample and Hold/1 -> Subtract/2
  Logical Operator1/1 -> Sample and Hold1/Trigger
  Delay1/1 -> Logical Operator2/1
  In1/1 -> Logical Operator1/1, Delay1/1, Delay2/1, Logical Operator4/1
  [on_time] -> Subtract1/2
  on? (I/O)3/1 -> Switch2/1
  Sample and Hold1/1 -> [on_time], Scope20/1, Subtract/1
  on? (I/O)7/1 -> Switch4/3
  Delay2/1 -> Logical Operator3/2
  Logical Operator2/1 -> Logical Operator1/2
  Switch4/1 -> Switch3/1
  Logical Operator3/1 -> Sample and Hold/Trigger
  Clock/1 -> Sample and Hold1/1
  Logical Operator4/1 -> Logical Operator3/1
  on? (I/O)6/1 -> Switch4/1
  Subtract1/1 -> Switch4/2
  Subtract/1 -> Switch2/2
  on? (I/O)5/1 -> Switch3/3
  Memory/1 -> Out1/1
  Switch3/1 -> Memory/1
  on? (I/O)4/1 -> Switch2/3
  Clock1/1 -> Subtract1/1
  Ground/1 -> Scope20/2
  Switch2/1 -> Scope21/1, Switch3/2

== system Final_EWASP_VC/Subsystem3 ==
  note: roof masses (45kg/m^2) and heat capacities calculated
      | using https://www.steelbeamcalculator.co.uk/standardloads
  In1 : Inport
  In2 : Inport  Port=2
  In3 : Inport  Port=3
  Ceil node tmperatures : DiscreteIntegrator  InitialConditionSource=external  InitialCondition=20  SampleTime=-1  ICPrevOutput=DiscIntNeverNeededParam  ICPrevScaledInput=DiscIntNeverNeededParam
  Display1 : Display
  Divide : Product  Inputs=*/
  Divide1 : Product  Inputs=*/
  Heat to ceilingNodes : Product  Inputs=4
  Heat to roofspace airnode : Sum  Inputs=+
  Heatloss roof to environment : Subsystem
  MATLAB Function1 : MATLAB Function  TreatAsAtomicUnit=on
  MATLAB Function2 : MATLAB Function  TreatAsAtomicUnit=on
  MATLAB Function3 : MATLAB Function  TreatAsAtomicUnit=on
  MATLAB Function4 : MATLAB Function  TreatAsAtomicUnit=on
  Product1 : Product  Inputs=3
  "Roof Temp " : DiscreteIntegrator  InitialConditionSource=external  InitialCondition=20  SampleTime=-1  ICPrevOutput=DiscIntNeverNeededParam  ICPrevScaledInput=DiscIntNeverNeededParam
  "RoofspaceTemp " : DiscreteIntegrator  InitialConditionSource=external  InitialCondition=20  SampleTime=-1  ICPrevOutput=DiscIntNeverNeededParam  ICPrevScaledInput=DiscIntNeverNeededParam
  Subtract : Sum  Inputs=+-
  Subtract1 : Sum
  Subtract2 : Sum  Inputs=+-
  Subtract3 : Sum  Inputs=+-
  Subtract4 : Sum  Inputs=2
  Subtract5 : Sum  Inputs=-+
  Total roofstructure heat capacity : Product
  Unary Minus : UnaryMinus
  air density per m3 : Constant  Value=1.225
  air heat capacity per kg : Constant  Value=1000
  ceiling heatchange due to loss to roofspace : UnaryMinus
  ceilnode heat capacities(predominantly plaster mass) : Constant  Value=10*1090*(IsTop(1:1:11)').*floorOrCeilingArea(1:1:11)'
  ceilnode heat capacities(predominantly plaster mass)1 : Constant  Value=10*1090*(IsTop(1,1:11)').*floorOrCeilingArea(1,1:11)'
  convective transfer to ceiling node : Constant  Value=2
  deltaTCeilingNodes : Product  Inputs=*/
  deltaTCeilingNodes1 : Product  Inputs=*/
  estimate of pitched roofspace air volume: 0.5 * floorArea of loft * height at peak : Constant  Value=0.5*sum(floorOrCeilingArea(1,1:11)'.*IsTop(1,1:11)')*(0.5*(sum(floorOrCeilingArea(1,1:11)'.*IsTop(1,1:11)')).^0.5)
  heat loss ceiing to roofspace : Product
  heat loss roofspace to roof : Product
  initial ceilnode temps : Constant  Value=20*ones(11,1)
  initial ceilnode temps1 : Constant  Value=10
  initial ceilnode temps2 : Constant  Value=10
  mass of roof per m^2*predictedroofarea : Constant  Value=45*sum(floorOrCeilingArea(1,1:11)'.*IsTop(1,1:11)')*1.414
  roofspace heatchange due to loss to roof : UnaryMinus
  room is on the top floor : Constant  Value=IsTop(1,1:11)'
  room is on the top floor1 : Constant  Value=floorOrCeilingArea(1,1:11)'
  slate heat capacity per kg1 : Constant  Value=760
  w/k loss from ceiling to roofspace : Constant  Value=(ceilingU*2)*(floorOrCeilingArea(1,1:11)').*(IsTop(1,1:11)')
  w/k loss from roofspace to roof : Constant  Value=(ceilingU*2)*sum(floorOrCeilingArea(1,1:11)'.*IsTop(1,1:11)')*1.414
  Out1 : Outport  VectorParamsAs1DForOutWhenUnconnected=off
  wires:
  In2/1 -> [windSpeed]
  In1/1 -> Subtract/1
  Subtract5/1 -> Divide1/1
  w/k loss from roofspace to roof/1 -> heat loss roofspace to roof/2
  Subtract/1 -> Heat to ceilingNodes/1
  Product1/1 -> Divide/2
  estimate of pitched roofspace air volume: 0.5 * floorArea of loft * height at peak/1 -> Product1/2
  air heat capacity per kg/1 -> Product1/3
  room is on the top floor/1 -> Heat to ceilingNodes/2
  heat loss roofspace to roof/1 -> roofspace heatchange due to loss to roof/1, Subtract5/2
  MATLAB Function3/1(y) -> Subtract1/2
  convective transfer to ceiling node/1 -> Heat to ceilingNodes/4
  air density per m3/1 -> Product1/1
  initial ceilnode temps1/1 -> "RoofspaceTemp "/2
  Heatloss roof to environment/1(Out1) -> Subtract5/1
  Heat to roofspace airnode/1 -> Display1/1, Subtract4/1
  Total roofstructure heat capacity/1 -> Divide1/2
  slate heat capacity per kg1/1 -> Total roofstructure heat capacity/1
  deltaTCeilingNodes1/1 -> MATLAB Function3/1(u)
  ceilnode heat capacities(predominantly plaster mass)1/1 -> deltaTCeilingNodes1/2
  MATLAB Function4/1(y) -> "Roof Temp "/1
  w/k loss from ceiling to roofspace/1 -> heat loss ceiing to roofspace/2
  deltaTCeilingNodes/1 -> MATLAB Function1/1(u)
  Subtract4/1 -> Divide/1
  Subtract3/1 -> heat loss roofspace to roof/1
  MATLAB Function2/1(y) -> "RoofspaceTemp "/1
  room is on the top floor1/1 -> Heat to ceilingNodes/3
  Ceil node tmperatures/1 -> Subtract2/1, Subtract/2
  mass of roof per m^2*predictedroofarea/1 -> Total roofstructure heat capacity/2
  ceilnode heat capacities(predominantly plaster mass)/1 -> deltaTCeilingNodes/2
  ceiling heatchange due to loss to roofspace/1 -> deltaTCeilingNodes1/1
  [windSpeed] -> Heatloss roof to environment/1(In1)
  initial ceilnode temps2/1 -> "Roof Temp "/2
  Heat to ceilingNodes/1 -> Unary Minus/1, deltaTCeilingNodes/1
  MATLAB Function1/1(y) -> Subtract1/1
  In3/1 -> [outdoorTemp]
  roofspace heatchange due to loss to roof/1 -> Subtract4/2
  Subtract2/1 -> heat loss ceiing to roofspace/1
  Divide1/1 -> MATLAB Function4/1(u)
  Divide/1 -> MATLAB Function2/1(u)
  "RoofspaceTemp "/1 -> Subtract3/1, Subtract2/2
  [outdoorTemp] -> Heatloss roof to environment/2(In2)
  Subtract1/1 -> Ceil node tmperatures/1
  initial ceilnode temps/1 -> Ceil node tmperatures/2
  heat loss ceiing to roofspace/1 -> ceiling heatchange due to loss to roofspace/1, Heat to roofspace airnode/1
  "Roof Temp "/1 -> Subtract3/2, Heatloss roof to environment/3(In3)
  Unary Minus/1 -> Out1/1

== system Final_EWASP_VC/Subsystem4 ==
  In1 : Inport
  Constant13 : Constant  Value=5
  "Select correct element from array, considering offset6" : Subsystem
  multiplication accounts for input data # being scaled 5 times too small : Product  Inputs=**
  Out1 : Outport  VectorParamsAs1DForOutWhenUnconnected=off
  wires:
  "Select correct element from array, considering offset6"/1(Out1) -> multiplication accounts for input data # being scaled 5 times too small/1
  In1/1 -> "Select correct element from array, considering offset6"/1(In1)
  Constant13/1 -> multiplication accounts for input data # being scaled 5 times too small/2
  multiplication accounts for input data # being scaled 5 times too small/1 -> Out1/1

== system Final_EWASP_VC/Subsystem_Room1 ==
  DNI1 : Constant  Value=50
  Diffuse Irradiance1 : Constant  Value=50
  Ground : Ground
  Incidence Angle1 : Constant  Value=60
  Integrator : Integrator  InitialConditionSource=external  InitialCondition=Tin1
  Lounge/Dining : Subsystem
      mask Display:
      | port_label('input', 1, 'THB in')
      | port_label('input', 2, 'Mdot_Rad_Full_open')
      | port_label('input', 3, 'T In')
      | port_label('input', 4, 'T Out')
      | port_label('input', 5, 'T up (conv)')
      | port_label('input', 6, 'T Down (conv)')
      | port_label('input', 7, 'T Bel (cond)')
      | port_label('input', 8, 'T Abv (cond)')
      | port_label('input', 9, 'T N1')
      | port_label('input', 10, 'T N2')
      | port_label('input', 11, 'T N3')
      | port_label('input', 12, 'T N4')
      | port_label('input', 13, 'T N5')
      | port_label('input', 14, 'T Wall')
      | port_label('input', 15, 'Ang')
      | port_label('input', 16, 'Tilt')
      | port_label('input', 17, 'DNI')
      | port_label('input', 18, 'DiffI')
      | 
      | port_label('output', 1, 'THB Out')
      | port_label('output', 2, 'DeltaT Wall')
      | port_label('output', 3, 'DeltaT Room')
      | port_label('output', 5, 'Mdot_Actual')
  Panel TIlt1 : Constant  Value=90
  Scope : Scope
  Subsystem11 : Subsystem
      mask Display:
      | disp('Vertical \n Conductive \n Signalling \n Block')
      | port_label('input', 1, 'Bel1')
      | port_label('input', 2, 'Bel2')
      | port_label('input', 3, 'Abv1')
      | port_label('input', 4, 'Abv2')
      | 
      | port_label('output', 1, 'T Bel')
      | port_label('output', 2, 'T Abv')
  Subsystem3 : Subsystem
      mask Display:
      | disp('Horizontal \n Neighbour \n Signalling \n Block')
      | port_label('input', 1, 'Nbr1')
      | port_label('input', 2, 'Nbr2')
      | port_label('input', 3, 'Nbr3')
      | port_label('input', 4, 'Nbr4')
      | port_label('input', 5, 'Nbr5')
      | port_label('output', 1, 'TN1')
      | port_label('output', 2, 'TN2')
      | port_label('output', 3, 'TN3')
      | port_label('output', 4, 'TN4')
      | port_label('output', 5, 'TN5')
  Terminator14 : Terminator
  Terminator2 : Terminator
  Tinitial1 : Constant  Value=21
  Twall11 : Constant  Value=neighbourMatrix(1,1)
  Twall12 : Constant  Value=neighbourMatrix(2,1)
  Twall13 : Constant  Value=neighbourMatrix(3,1)
  Twall14 : Constant  Value=neighbourMatrix(4,1)
  Twall15 : Constant  Value=neighbourMatrix(5,1)
  Twall33 : Constant  Value=condUDMatrix(1,1)
  Twall34 : Constant  Value=condUDMatrix(2,1)
  Twall35 : Constant  Value=condUDMatrix(3,1)
  Twall36 : Constant  Value=condUDMatrix(4,1)
  tag scope: DeltaT_1=global, Mdot_Actual_1=global, T_1=global, T_return_R1=global
  wires:
  [T_Out] -> Lounge/Dining/4(In3)
  Subsystem11/1(Out1) -> Lounge/Dining/7(In6)
  [T_1] -> Lounge/Dining/3(In2)
  Incidence Angle1/1 -> Lounge/Dining/15(In14)
  DNI1/1 -> Lounge/Dining/17(In16)
  Twall34/1 -> Subsystem11/2(In2)
  Subsystem3/5(Out5) -> Lounge/Dining/13(In12)
  Twall36/1 -> Subsystem11/4(In4)
  Twall33/1 -> Subsystem11/1(In1)
  Tinitial1/1 -> Integrator/2
  [DeltaT_1] -> Scope/1, Integrator/1
  [T_1] -> Lounge/Dining/5(In4), Lounge/Dining/6(In5)
  Twall11/1 -> Subsystem3/1(In1)
  Lounge/Dining/5(Out5) -> [Mdot_Actual_1]
  Subsystem3/1(Out1) -> Lounge/Dining/9(In8)
  Lounge/Dining/3(Out3) -> [DeltaT_1]
  Lounge/Dining/1(Out1) -> [T_return_R1]
  Lounge/Dining/4(Out4) -> Terminator2/1
  Diffuse Irradiance1/1 -> Lounge/Dining/18(In17)
  Lounge/Dining/2(Out2) -> Terminator14/1
  [THB_In] -> Lounge/Dining/1(In1)
  [MassFlow_Full_Open_1] -> Lounge/Dining/2(In18)
  Subsystem3/4(Out4) -> Lounge/Dining/12(In11)
  Twall13/1 -> Subsystem3/3(In3)
  Subsystem3/3(Out3) -> Lounge/Dining/11(In10)
  Twall15/1 -> Subsystem3/5(In5)
  Subsystem11/2(Out2) -> Lounge/Dining/8(In7)
  Ground/1 -> Lounge/Dining/14(In13)
  Twall14/1 -> Subsystem3/4(In4)
  Panel TIlt1/1 -> Lounge/Dining/16(In15)
  Integrator/1 -> [T_1]
  Twall12/1 -> Subsystem3/2(In2)
  Subsystem3/2(Out2) -> Lounge/Dining/10(In9)
  Twall35/1 -> Subsystem11/3(In3)

== system Final_EWASP_VC/Subsystem_Room10 ==
  DNI15 : Constant  Value=0
  Diffuse Irradiance10 : Constant  Value=0
  En suite : Subsystem
      mask Display:
      | port_label('input', 1, 'THB in')
      | port_label('input', 2, 'T In')
      | port_label('input', 3, 'T Out')
      | port_label('input', 4, 'T up (conv)')
      | port_label('input', 5, 'T Down (conv)')
      | port_label('input', 6, 'T Bel (cond)')
      | port_label('input', 7, 'T Abv (cond)')
      | port_label('input', 8, 'T N1')
      | port_label('input', 9, 'T N2')
      | port_label('input', 10, 'T N3')
      | port_label('input', 11, 'T N4')
      | port_label('input', 12, 'T N5')
      | port_label('input', 13, 'T Wall')
      | port_label('input', 14, 'Ang')
      | port_label('input', 15, 'Tilt')
      | port_label('input', 16, 'DNI')
      | port_label('input', 17, 'DiffI')
      | 
      | port_label('output', 1, 'THB Out')
      | port_label('output', 2, 'DeltaT Wall')
      | port_label('output', 3, 'DeltaT Room')
      | 
      | port_label('input', 18, 'm_dot_Fully_open')
      | port_label('output', 5, 'm_dot_Actual')
  Ground6 : Ground
  Incidence Angle10 : Constant  Value=60
  Integrator20 : Integrator  InitialConditionSource=external  InitialCondition=Tin1
  Panel TIlt10 : Constant  Value=90
  Scope34 : Scope
  Subsystem12 : Subsystem
      mask Display:
      | disp('Horizontal \n Neighbour \n Signalling \n Block')
      | port_label('input', 1, 'Nbr1')
      | port_label('input', 2, 'Nbr2')
      | port_label('input', 3, 'Nbr3')
      | port_label('input', 4, 'Nbr4')
      | port_label('input', 5, 'Nbr5')
      | port_label('output', 1, 'TN1')
      | port_label('output', 2, 'TN2')
      | port_label('output', 3, 'TN3')
      | port_label('output', 4, 'TN4')
      | port_label('output', 5, 'TN5')
  Subsystem23 : Subsystem
      mask Display:
      | disp('Vertical \n Convective \n Signalling \n Block')
      | port_label('input', 1, 'Nbr1')
      | port_label('input', 2, 'Nbr2')
      | 
      | port_label('output', 1, 'Tup')
      | port_label('output', 2, 'Tdwn')
  Subsystem28 : Subsystem
      mask Display:
      | disp('Vertical \n Conductive \n Signalling \n Block')
      | port_label('input', 1, 'Bel1')
      | port_label('input', 2, 'Bel2')
      | port_label('input', 3, 'Abv1')
      | port_label('input', 4, 'Abv2')
      | 
      | port_label('output', 1, 'T Bel')
      | port_label('output', 2, 'T Abv')
  Terminator7 : Terminator
  Tinitial14 : Constant  Value=20
  Twall100 : Constant  Value=condUDMatrix(1,10)
  Twall101 : Constant  Value=condUDMatrix(2,10)
  Twall102 : Constant  Value=condUDMatrix(3,10)
  Twall103 : Constant  Value=condUDMatrix(4,10)
  Twall51 : Constant  Value=neighbourMatrix(1,10)
  Twall52 : Constant  Value=neighbourMatrix(2,10)
  Twall53 : Constant  Value=neighbourMatrix(3,10)
  Twall54 : Constant  Value=neighbourMatrix(4,10)
  Twall55 : Constant  Value=neighbourMatrix(5,10)
  Twall82 : Constant  Value=convUDMatrix(1,10)
  Twall83 : Constant  Value=convUDMatrix(2,10)
  tag scope: DeltaT_10=global, Mdot_Actual_10=global, T_10=global, T_return_R10=global
  wires:
  Tinitial14/1 -> Integrator20/2
  [DeltaT_10] -> Integrator20/1
  Ground6/1 -> En suite/13(In13)
  Subsystem12/1(Out1) -> En suite/8(In8)
  [MassFlow_Full_Open_10] -> En suite/18(In18)
  DNI15/1 -> En suite/16(In16)
  Twall82/1 -> Subsystem23/1(In1)
  Subsystem12/4(Out4) -> En suite/11(In11)
  Panel TIlt10/1 -> En suite/15(In15)
  Subsystem28/2(Out2) -> En suite/7(In7)
  Twall55/1 -> Subsystem12/5(In5)
  [THB_In] -> En suite/1(In1)
  Diffuse Irradiance10/1 -> En suite/17(In17)
  En suite/3(Out3) -> [DeltaT_10]
  Twall83/1 -> Subsystem23/2(In2)
  En suite/2(Out2) -> Terminator7/1
  En suite/5(Out5) -> [Mdot_Actual_10]
  En suite/1(Out1) -> [T_return_R10]
  Incidence Angle10/1 -> En suite/14(In14)
  Twall102/1 -> Subsystem28/3(In3)
  [T_10] -> En suite/2(In2)
  Twall53/1 -> Subsystem12/3(In3)
  Integrator20/1 -> [T_10]
  Subsystem12/2(Out2) -> En suite/9(In9)
  Subsystem23/2(Out2) -> En suite/5(In5)
  Subsystem12/3(Out3) -> En suite/10(In10)
  En suite/4(Out4) -> Scope34/1
  Subsystem23/1(Out1) -> En suite/4(In4)
  Twall54/1 -> Subsystem12/4(In4)
  Twall100/1 -> Subsystem28/1(In1)
  Subsystem12/5(Out5) -> En suite/12(In12)
  Twall52/1 -> Subsystem12/2(In2)
  [T_Out] -> En suite/3(In3)
  Twall103/1 -> Subsystem28/4(In4)
  Twall51/1 -> Subsystem12/1(In1)
  Subsystem28/1(Out1) -> En suite/6(In6)
  Twall101/1 -> Subsystem28/2(In2)

== system Final_EWASP_VC/Subsystem_Room11 ==
  Bathroom : Subsystem
      mask Display:
      | port_label('input', 1, 'THB in')
      | port_label('input', 2, 'T In')
      | port_label('input', 3, 'T Out')
      | port_label('input', 4, 'T up (conv)')
      | port_label('input', 5, 'T Down (conv)')
      | port_label('input', 6, 'T Bel (cond)')
      | port_label('input', 7, 'T Abv (cond)')
      | port_label('input', 8, 'T N1')
      | port_label('input', 9, 'T N2')
      | port_label('input', 10, 'T N3')
      | port_label('input', 11, 'T N4')
      | port_label('input', 12, 'T N5')
      | port_label('input', 13, 'T Wall')
      | port_label('input', 14, 'Ang')
      | port_label('input', 15, 'Tilt')
      | port_label('input', 16, 'DNI')
      | port_label('input', 17, 'DiffI')
      | 
      | port_label('output', 1, 'THB Out')
      | port_label('output', 2, 'DeltaT Wall')
      | port_label('output', 3, 'DeltaT Room')
      | 
      | port_label('input', 18, 'm_dot_Fully_open')
      | port_label('output', 5, 'm_dot_Actual')
  DNI9 : Constant  Value=0
  Diffuse Irradiance11 : Constant  Value=0
  Ground5 : Ground
  Incidence Angle11 : Constant  Value=60
  Integrator24 : Integrator  InitialConditionSource=external  InitialCondition=Tin1
  Panel TIlt11 : Constant  Value=90
  Scope33 : Scope
  Subsystem13 : Subsystem
      mask Display:
      | disp('Horizontal \n Neighbour \n Signalling \n Block')
      | port_label('input', 1, 'Nbr1')
      | port_label('input', 2, 'Nbr2')
      | port_label('input', 3, 'Nbr3')
      | port_label('input', 4, 'Nbr4')
      | port_label('input', 5, 'Nbr5')
      | port_label('output', 1, 'TN1')
      | port_label('output', 2, 'TN2')
      | port_label('output', 3, 'TN3')
      | port_label('output', 4, 'TN4')
      | port_label('output', 5, 'TN5')
  Subsystem24 : Subsystem
      mask Display:
      | disp('Vertical \n Convective \n Signalling \n Block')
      | port_label('input', 1, 'Nbr1')
      | port_label('input', 2, 'Nbr2')
      | 
      | port_label('output', 1, 'Tup')
      | port_label('output', 2, 'Tdwn')
  Subsystem29 : Subsystem
      mask Display:
      | disp('Vertical \n Conductive \n Signalling \n Block')
      | port_label('input', 1, 'Bel1')
      | port_label('input', 2, 'Bel2')
      | port_label('input', 3, 'Abv1')
      | port_label('input', 4, 'Abv2')
      | 
      | port_label('output', 1, 'T Bel')
      | port_label('output', 2, 'T Abv')
  Terminator8 : Terminator
  Tinitial15 : Constant  Value=20
  Twall123 : Constant  Value=condUDMatrix(1,11)
  Twall133 : Constant  Value=condUDMatrix(2,11)
  Twall134 : Constant  Value=condUDMatrix(3,11)
  Twall135 : Constant  Value=condUDMatrix(4,11)
  Twall56 : Constant  Value=neighbourMatrix(1,11)
  Twall57 : Constant  Value=neighbourMatrix(2,11)
  Twall58 : Constant  Value=neighbourMatrix(3,11)
  Twall59 : Constant  Value=neighbourMatrix(4,11)
  Twall60 : Constant  Value=neighbourMatrix(5,11)
  Twall84 : Constant  Value=convUDMatrix(1,11)
  Twall85 : Constant  Value=convUDMatrix(2,11)
  tag scope: DeltaT_11=global, Mdot_Actual_11=global, T_11=global, T_return_R11=global
  wires:
  Bathroom/1(Out1) -> [T_return_R11]
  [DeltaT_11] -> Integrator24/1
  [MassFlow_Full_Open_11] -> Bathroom/18(In18)
  Diffuse Irradiance11/1 -> Bathroom/17(In17)
  Subsystem13/1(Out1) -> Bathroom/8(In8)
  Subsystem13/3(Out3) -> Bathroom/10(In10)
  Subsystem13/2(Out2) -> Bathroom/9(In9)
  Subsystem24/2(Out2) -> Bathroom/5(In5)
  Bathroom/4(Out4) -> Scope33/1
  Subsystem13/4(Out4) -> Bathroom/11(In11)
  [T_11] -> Bathroom/2(In2)
  Twall57/1 -> Subsystem13/2(In2)
  Bathroom/3(Out3) -> [DeltaT_11]
  DNI9/1 -> Bathroom/16(In16)
  Twall58/1 -> Subsystem13/3(In3)
  Twall135/1 -> Subsystem29/4(In4)
  Twall84/1 -> Subsystem24/1(In1)
  Twall59/1 -> Subsystem13/4(In4)
  Tinitial15/1 -> Integrator24/2
  Twall123/1 -> Subsystem29/1(In1)
  Panel TIlt11/1 -> Bathroom/15(In15)
  Twall60/1 -> Subsystem13/5(In5)
  Subsystem24/1(Out1) -> Bathroom/4(In4)
  Twall85/1 -> Subsystem24/2(In2)
  Integrator24/1 -> [T_11]
  [T_Out] -> Bathroom/3(In3)
  Subsystem29/2(Out2) -> Bathroom/7(In7)
  Twall56/1 -> Subsystem13/1(In1)
  Bathroom/2(Out2) -> Terminator8/1
  [THB_In] -> Bathroom/1(In1)
  Bathroom/5(Out5) -> [Mdot_Actual_11]
  Twall134/1 -> Subsystem29/3(In3)
  Subsystem13/5(Out5) -> Bathroom/12(In12)
  Incidence Angle11/1 -> Bathroom/14(In14)
  Twall133/1 -> Subsystem29/2(In2)
  Subsystem29/1(Out1) -> Bathroom/6(In6)
  Ground5/1 -> Bathroom/13(In13)
